simulink model "simulateDSSS_binaryMessage_withTS"  (R2017a)
settings: Solver=VariableStepAuto  StartTime=0.0  StopTime=10  RelTol=1e-3
InitFcn:
  | Tb = .1;
  | Tc = 0.01;
  | fs = 1e3;
  | Ts = 1/fs;
libraries: commfilt2 x4, dspsrcs4 x2, commchan3 x1, commdigbbndpm3 x1, commrandsrc3 x1
settings Model: Creator=prust  LastModifiedBy=prust

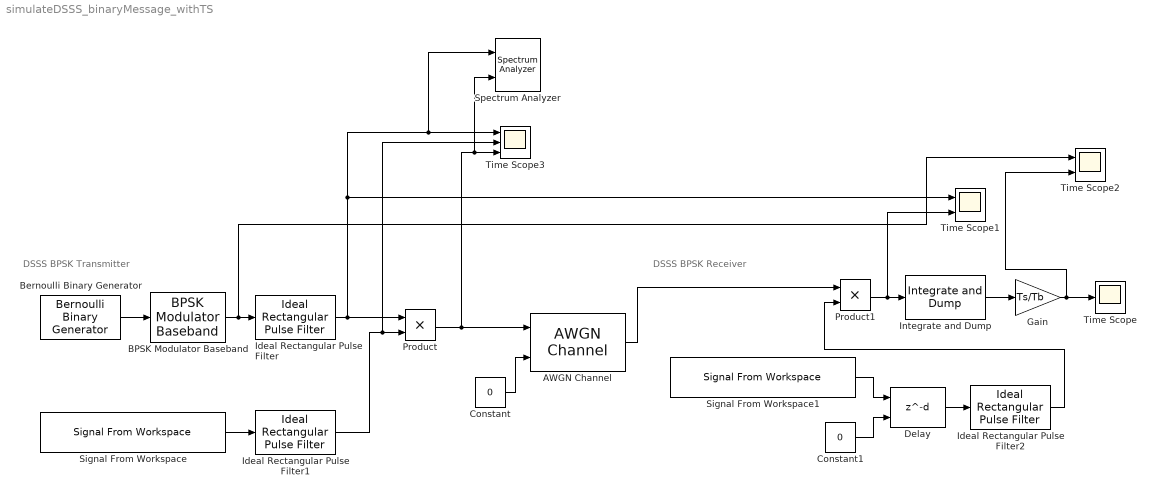
== system simulateDSSS_binaryMessage_withTS ==
  note: DSSS BPSK Transmitter
  note: DSSS BPSK Receiver
  AWGN Channel : commchan3/AWGN Channel  InputProcessing=Columns as channels (frame based)  seed=67  noiseMode=Variance from port  EbNodB=10  EsNodB=10  SNRdB=10  bitsPerSym=1  Ps=1  Tsym=1  variance=1
  BPSK Modulator Baseband : commdigbbndpm3/BPSK Modulator Baseband  Ph=0  outDtype=double  outWordLen=16  outUDDataType=sfix(16)  outFracLenMode=Best precision  outFracLen=15  outDataTypeStr=double  outLastDataTypeStr=double
  Bernoulli Binary Generator : commrandsrc3/Bernoulli Binary Generator  ProbabilityOfZero=0.5  SeedSource=Auto  Seed=0  SampleTime=Tb  SamplesPerFrame=100  OutputDataType=double  SimulateUsing=Interpreted execution
  Constant : Constant  Value=0
  Constant1 : Constant  Value=0
  Delay : Delay  DelayLengthSource=Input port  DelayLength=1  InputProcessing=Columns as channels (frame based)
      settings: InputPortMap=u0,p1
  Gain : Gain  Gain=Ts/Tb
  Ideal Rectangular Pulse Filter : commfilt2/Ideal Rectangular Pulse Filter  pulseLen=Tb/Ts  pulseDelay=0  InputProcessing=Columns as channels (frame based)  RateOptions=Allow multirate processing  sampMode=Mute  normCheck=off  normMode=Sum of samples  filterGain=1  saveAsFlag=0  roundingMode=Floor  overflowMode=off  firstCoeffDataTypeStr=Inherit: Same word length as input  firstCoeffMin=[]  firstCoeffMax=[]  firstCoeffLastDataTypeStr=Inherit: Same word length as input  outputDataTypeStr=Inherit: Same as accumulator  outputMin=[]  outputMax=[]  outputLastDataTypeStr=Inherit: Same as accumulator
      settings: SourceProductName=Communications System Toolbox  SourceProductBaseCode=CM
  Ideal Rectangular Pulse Filter1 : commfilt2/Ideal Rectangular Pulse Filter  pulseLen=Tc/Ts  pulseDelay=0  InputProcessing=Columns as channels (frame based)  RateOptions=Allow multirate processing  sampMode=Mute  normCheck=off  normMode=Sum of samples  filterGain=1  saveAsFlag=0  roundingMode=Floor  overflowMode=off  firstCoeffDataTypeStr=Inherit: Same word length as input  firstCoeffMin=[]  firstCoeffMax=[]  firstCoeffLastDataTypeStr=Inherit: Same word length as input  outputDataTypeStr=Inherit: Same as accumulator  outputMin=[]  outputMax=[]  outputLastDataTypeStr=Inherit: Same as accumulator
      settings: SourceProductName=Communications System Toolbox  SourceProductBaseCode=CM
  Ideal Rectangular Pulse Filter2 : commfilt2/Ideal Rectangular Pulse Filter  pulseLen=Tc/Ts  pulseDelay=0  InputProcessing=Columns as channels (frame based)  RateOptions=Allow multirate processing  sampMode=Mute  normCheck=off  normMode=Sum of samples  filterGain=1  saveAsFlag=0  roundingMode=Floor  overflowMode=off  firstCoeffDataTypeStr=Inherit: Same word length as input  firstCoeffMin=[]  firstCoeffMax=[]  firstCoeffLastDataTypeStr=Inherit: Same word length as input  outputDataTypeStr=Inherit: Same as accumulator  outputMin=[]  outputMax=[]  outputLastDataTypeStr=Inherit: Same as accumulator
      settings: SourceProductName=Communications System Toolbox  SourceProductBaseCode=CM
  Integrate and Dump : commfilt2/Integrate and Dump  obssamples=Tb/Ts  offsetsamples=0  nodump=off  roundingMode=Floor  overflowMode=off  outputDataTypeStr=Inherit: Same as accumulator  outputLastDataTypeStr=Inherit: Same as accumulator
      settings: SourceProductName=Communications System Toolbox
  Product : Product
  Product1 : Product
  Signal From Workspace : dspsrcs4/Signal From Workspace  X=[-1 1 -1 1 1 1 -1 1 1 -1 -1 -1 1 1 1 1]  Ts=Tc  nsamps=100  OutputAfterFinalValue=Cyclic repetition  ignoreOrWarnInputAndFrameLengths=off  OutputFrames=off
  Signal From Workspace1 : dspsrcs4/Signal From Workspace  X=[-1 1 -1 1 1 1 -1 1 1 -1 -1 -1 1 1 1 1]  Ts=Tc  nsamps=100  OutputAfterFinalValue=Cyclic repetition  ignoreOrWarnInputAndFrameLengths=off  OutputFrames=off
  Spectrum Analyzer : SpectrumAnalyzer  NumInputPorts=2
  Time Scope : Scope
  Time Scope1 : Scope  NumInputPorts=2
  Time Scope2 : Scope  NumInputPorts=2
  Time Scope3 : Scope  NumInputPorts=3
  wires:
  Bernoulli Binary Generator/1 -> BPSK Modulator Baseband/1
  Constant/1 -> AWGN Channel/2
  Signal From Workspace1/1 -> Delay/1
  Delay/1 -> Ideal Rectangular Pulse Filter2/1
  Constant1/1 -> Delay/2
  Product/1 -> AWGN Channel/1, Spectrum Analyzer/2, Time Scope3/3
  AWGN Channel/1 -> Product1/1
  Ideal Rectangular Pulse Filter/1 -> Spectrum Analyzer/1, Time Scope3/1, Time Scope1/1, Product/1
  Ideal Rectangular Pulse Filter2/1 -> Product1/2
  Ideal Rectangular Pulse Filter1/1 -> Time Scope3/2, Product/2
  Signal From Workspace/1 -> Ideal Rectangular Pulse Filter1/1
  Product1/1 -> Time Scope1/2, Integrate and Dump/1
  Integrate and Dump/1 -> Gain/1
  Gain/1 -> Time Scope2/2, Time Scope/1
  BPSK Modulator Baseband/1 -> Time Scope2/1, Ideal Rectangular Pulse Filter/1
